simulink model "p5"  (R2013a)
settings: Solver=ode45  StartTime=0.0  StopTime=10.0  RelTol=1e-3
values from neighbouring files (symbols this model uses):
  A = [0 0 1 0; 0 0 0 1; 0 566 -37 0; 0 -922 37 0]    [CEELab.m]    (also in ex1.m; ex11a.m; ex11b.m; ex2.m)
  b = [0 0 65 -65]'    [CEELab.m]    (also in ex1.m; ex11a.m; ex11b.m; ex3.m)
  c = [1 1 0 0]    [CEELab.m]    (also in ex11a.m; ex11b.m; ex2.m; ex3.m)
  K = (alphaK(2:5)-a(2:5))*inv(M)'*inv(CM)    [CEELab.m]    (also in ex11a.m; ex11b.m; ex4.m; labtotal.m = (alphac-a)*((M^-1)')*(C^-1))
  L = inv(OM)*inv(M)*(alphaL(2:5)-a(2:5))'    [CEELab.m]    (also in ex11a.m; ex11b.m; ex4.m; labtotal.m = (O^-1)*(M^-1)*(alphao-a)')
settings Model: Creator=Rui G  LastModifiedBy=Rui G

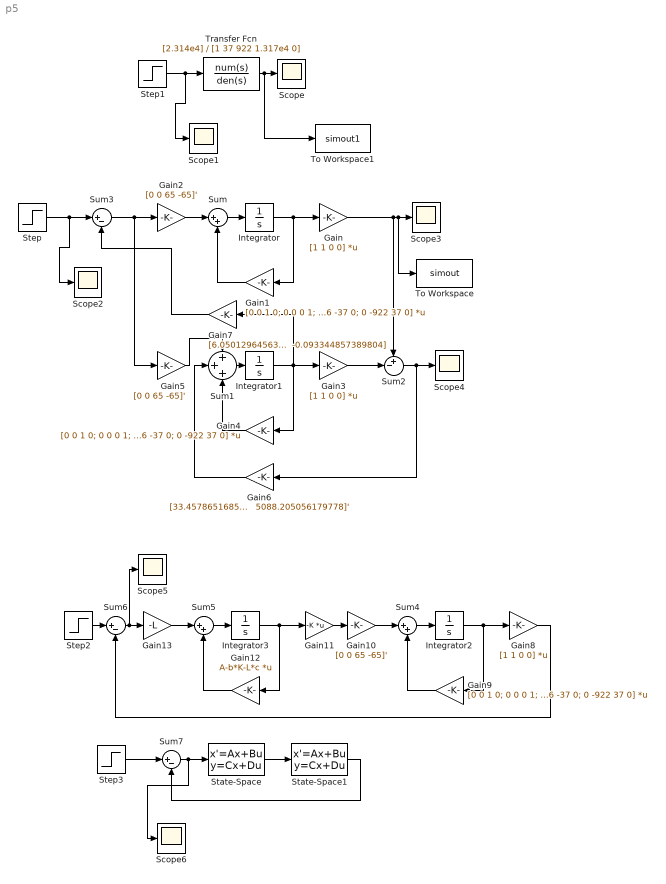
== system p5 ==
  Gain : Gain  Gain=[1 1 0 0]  Multiplication=Matrix(K*u) (u vector)
  Gain1 : Gain  Gain=[0 0 1 0; 0 0 0 1; 0 566 -37 0; 0 -922 37 0]  Multiplication=Matrix(K*u) (u vector)
  Gain10 : Gain  Gain=[0 0 65 -65]'
  Gain11 : Gain  Gain=-K  Multiplication=Matrix(K*u) (u vector)
  Gain12 : Gain  Gain=A-b*K-L*c  Multiplication=Matrix(K*u) (u vector)
  Gain13 : Gain  Gain=-L
  Gain2 : Gain  Gain=[0 0 65 -65]'
  Gain3 : Gain  Gain=[1 1 0 0]  Multiplication=Matrix(K*u) (u vector)
  Gain4 : Gain  Gain=[0 0 1 0; 0 0 0 1; 0 566 -37 0; 0 -922 37 0]  Multiplication=Matrix(K*u) (u vector)
  Gain5 : Gain  Gain=[0 0 65 -65]'
  Gain6 : Gain  Gain=|
      | [33.457865168539
      |    89.542134831461
      |   -1161.205056179773
      |    5088.205056179778]'
  Gain7 : Gain  Gain="[6.050129645635197 -30.534485738980159   1.029732065687119  -0.093344857389804]"
  Gain8 : Gain  Gain=[1 1 0 0]  Multiplication=Matrix(K*u) (u vector)
  Gain9 : Gain  Gain=[0 0 1 0; 0 0 0 1; 0 566 -37 0; 0 -922 37 0]  Multiplication=Matrix(K*u) (u vector)
  Integrator{,1..3} (4 alike) : Integrator
  Scope{,1..6} (7 alike) : Scope
      Scope settings: YMin=0  YMax=30000
      Scope2 settings: SaveName=ScopeData2
      Scope3 settings: YMin=0  YMax=30000  SaveName=ScopeData3
      Scope4 settings: YMin=0  YMax=30000  SaveName=ScopeData4
      Scope5 settings: SaveName=ScopeData5
      Scope6 settings: SaveName=ScopeData6
  State-Space : StateSpace  A=A-b*K-L*c  B=-L  C=-K  D=0
  State-Space1 : StateSpace  A=A  B=b  C=c  D=0
  Step{,1..3} (4 alike) : Step  Time=0  SampleTime=0
  Sum : Sum  Inputs=|++
  Sum1 : Sum  Inputs=+++
  Sum2 : Sum  Inputs=+-|
  Sum3 : Sum  Inputs=|+-
  Sum4 : Sum  Inputs=|++
  Sum5 : Sum  Inputs=|++
  Sum6 : Sum  Inputs=|+-
  Sum7 : Sum  Inputs=|+-
  To Workspace : ToWorkspace  VariableName=simout  SampleTime=-1  SaveFormat=Timeseries
  To Workspace1 : ToWorkspace  VariableName=simout1  SampleTime=-1  SaveFormat=Timeseries
  Transfer Fcn : TransferFcn  Numerator=[2.314e4]  Denominator=[1 37 922 1.317e4 0]
  wires:
  Step1/1 -> Scope1/1, Transfer Fcn/1
  Transfer Fcn/1 -> To Workspace1/1, Scope/1
  Gain2/1 -> Sum/1
  Sum/1 -> Integrator/1
  Integrator/1 -> Gain1/1, Gain/1
  Gain1/1 -> Sum/2
  Step/1 -> Sum3/1, Scope2/1
  Gain/1 -> Sum2/1, To Workspace/1, Scope3/1
  Gain5/1 -> Sum1/1
  Sum1/1 -> Integrator1/1
  Integrator1/1 -> Gain7/1, Gain4/1, Gain3/1
  Gain3/1 -> Sum2/2
  Gain4/1 -> Sum1/3
  Sum2/1 -> Scope4/1, Gain6/1
  Gain6/1 -> Sum1/2
  Sum3/1 -> Gain5/1, Gain2/1
  Gain7/1 -> Sum3/2
  Gain10/1 -> Sum4/1
  Sum4/1 -> Integrator2/1
  Integrator2/1 -> Gain9/1, Gain8/1
  Gain9/1 -> Sum4/2
  Gain13/1 -> Sum5/1
  Sum5/1 -> Integrator3/1
  Integrator3/1 -> Gain12/1, Gain11/1
  Gain12/1 -> Sum5/2
  Gain11/1 -> Gain10/1
  Sum6/1 -> Scope5/1, Gain13/1
  Gain8/1 -> Sum6/2
  Step2/1 -> Sum6/1
  State-Space/1 -> State-Space1/1
  Sum7/1 -> Scope6/1, State-Space/1
  State-Space1/1 -> Sum7/2
  Step3/1 -> Sum7/1
